simulink model "FlexibleJoint_ConventionalSMC"  (R2019b)
settings: Solver=VariableStepAuto  StartTime=0.0  StopTime=10.0  RelTol=1e-3
libraries: robotcorelib x1
settings Model: Creator=USER  LastModifiedBy=USER

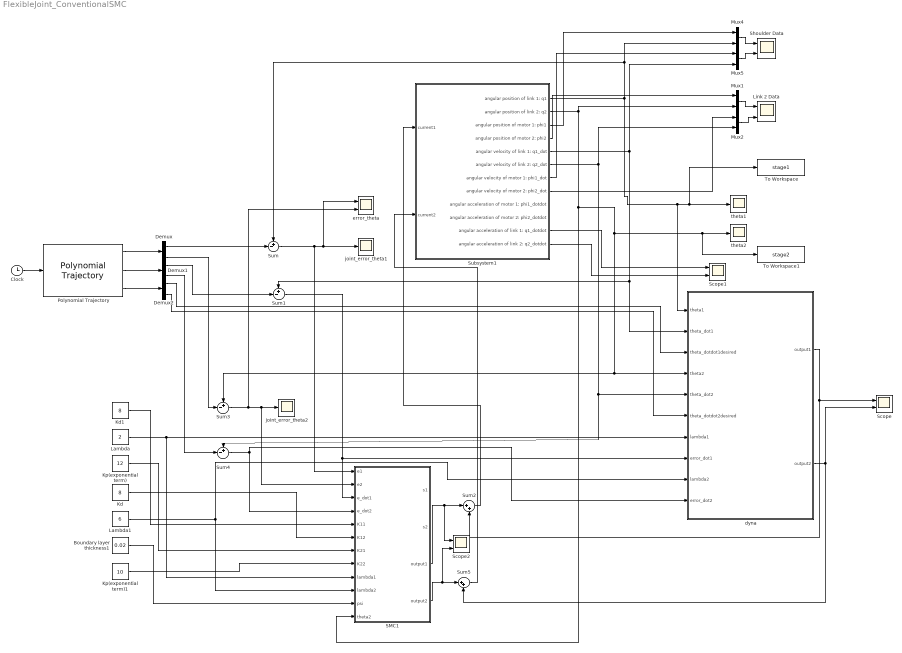
== system FlexibleJoint_ConventionalSMC ==
  Boundary layer thickness1 : Constant  Value=0.02
  Clock : Clock
  Demux : Demux  Outputs=2
  Demux1 : Demux  Outputs=2
  Demux2 : Demux  Outputs=2
  Kd : Constant  Value=8
  Kd1 : Constant  Value=8
  Kp(exponential term) : Constant  Value=12
  Kp(exponential term)1 : Constant  Value=10
  Lambda : Constant  Value=2
  Lambda1 : Constant  Value=6
  Link 2 Data : Scope  NumInputPorts=2
  Mux{1..2,4..5} (4 alike) : Mux  Inputs=2
  Polynomial Trajectory : robotcorelib/Polynomial Trajectory  WaypointSource=Internal  Waypoints=[ 0, pi/2; 0, pi/4]  TimePoints=[ 0, 5]  TimeInterval=[ 1, 4 ]  Method=Cubic Polynomial  ParameterSource=Internal  VelocityBoundaryCondition=zeros( 2, 2 )  AccelerationBoundaryCondition=zeros( 2, 5 )  SimulateUsing=Interpreted execution
      settings: SourceProductName=Robotics System Toolbox  SourceProductBaseCode=RO
  SMC1 : MATLAB Function  TreatAsAtomicUnit=on
  Scope : Scope  NumInputPorts=2
  Scope1 : Scope  NumInputPorts=2
  Scope2 : Scope  NumInputPorts=2
  Shoulder Data : Scope  NumInputPorts=2
  Subsystem1 : Subsystem
  Sum{,1,3..4} (4 alike) : Sum  Inputs=+-|
  Sum2 : Sum  Inputs=|++
  Sum5 : Sum  Inputs=|++
  To Workspace : ToWorkspace  VariableName=stage1  SaveFormat=Timeseries  SampleTime=-1
  To Workspace1 : ToWorkspace  VariableName=stage2  SaveFormat=Timeseries  SampleTime=-1
  dyna : MATLAB Function  TreatAsAtomicUnit=on
  error_theta : Scope  NumInputPorts=2
  joint_error_theta1 : Scope
  joint_error_theta2 : Scope
  theta1 : Scope
  theta2 : Scope
  wires:
  Subsystem1/5(angular velocity of link 1: q1_dot) -> Mux5/2, dyna/2(theta_dot1), Sum1/1
  Boundary layer thickness1/1 -> SMC1/11(psi)
  Sum1/1 -> SMC1/3(e_dot1), dyna/8(error_dot1)
  Sum4/1 -> dyna/10(error_dot2), SMC1/4(e_dot2)
  Polynomial Trajectory/1 -> Demux/1
  Subsystem1/12(angular acceleration of link 2: q2_dotdot) -> Scope1/2
  Demux1/2 -> Sum4/2
  Kp(exponential term)1/1 -> SMC1/8(K22)
  Clock/1 -> Polynomial Trajectory/1
  SMC1/3(output1) -> Scope2/1, Sum2/1
  Demux2/1 -> dyna/3(theta_dotdot1desired)
  Kd1/1 -> SMC1/5(K11)
  Lambda1/1 -> SMC1/10(lambda2), dyna/9(lambda2)
  Sum/1 -> SMC1/1(e1), joint_error_theta1/1, error_theta/1
  Demux1/1 -> Sum1/2
  Demux2/2 -> dyna/6(theta_dotdot2desired)
  Demux/1 -> Sum/2
  SMC1/4(output2) -> Scope2/2, Sum5/1
  Kp(exponential term)/1 -> SMC1/7(K21)
  Polynomial Trajectory/2 -> Demux1/1
  Sum2/1 -> Subsystem1/1(current1)
  Lambda/1 -> SMC1/9(lambda1), dyna/7(lambda1)
  Demux/2 -> Sum3/2
  dyna/2(output2) -> Scope/2, Sum5/2
  Subsystem1/2(angular position of link 2: q2) -> To Workspace1/1, theta2/1, Sum3/1, dyna/4(theta2), SMC1/12(theta2), Mux1/2
  Subsystem1/6(angular velocity of link 2: q2_dot) -> Sum4/1, dyna/5(theta_dot2), Mux2/2
  Polynomial Trajectory/3 -> Demux2/1
  Kd/1 -> SMC1/6(K12)
  Sum3/1 -> SMC1/2(e2), joint_error_theta2/1, error_theta/2
  Subsystem1/11(angular acceleration of link 1: q1_dotdot) -> Scope1/1
  dyna/1(output1) -> Scope/1, Sum2/2
  Sum5/1 -> Subsystem1/2("current2 ")
  Subsystem1/1(angular position of link 1: q1) -> Mux4/2, Sum/1, dyna/1(theta1), To Workspace/1, theta1/1
  Mux5/1 -> Shoulder Data/2
  Mux4/1 -> Shoulder Data/1
  Mux1/1 -> Link 2 Data/1
  Mux2/1 -> Link 2 Data/2
  Subsystem1/3(angular position of motor 1: phi1) -> Mux4/1
  Subsystem1/7(angular velocity of motor 1: phi1_dot) -> Mux5/1
  Subsystem1/4(angular position of motor 2: phi2) -> Mux1/1
  Subsystem1/8(angular velocity of motor 2: phi2_dot) -> Mux2/1

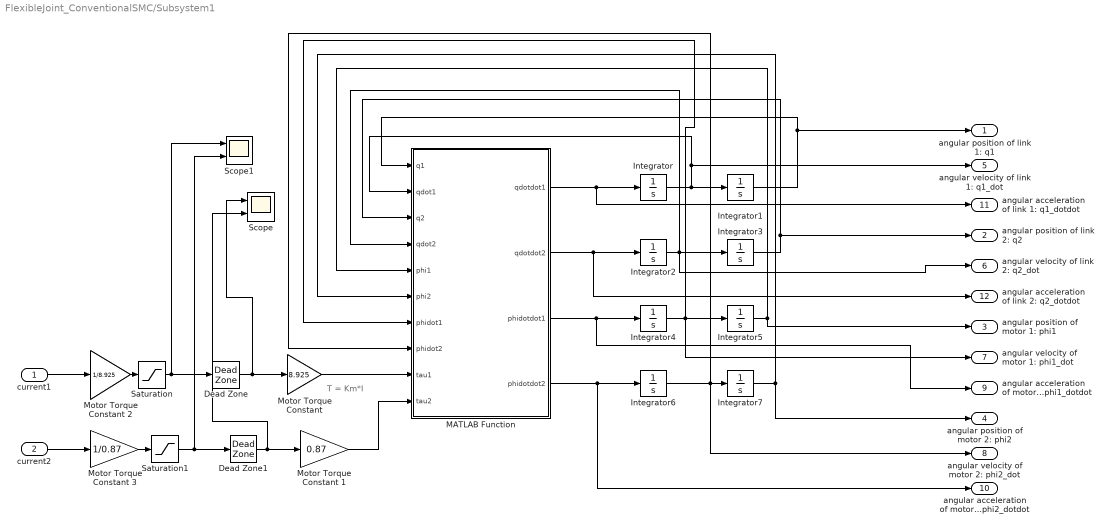
== system FlexibleJoint_ConventionalSMC/Subsystem1 ==
  note: T = Km*I
  current1 : Inport
  "current2 " : Inport  Port=2
  Dead Zone : DeadZone  LowerValue=-0.15  UpperValue=0.15  ZeroCross=off  SaturateOnIntegerOverflow=on
  Dead Zone1 : DeadZone  LowerValue=-0.15  UpperValue=0.15  ZeroCross=off  SaturateOnIntegerOverflow=on
  Integrator{,1..7} (8 alike) : Integrator
  MATLAB Function : MATLAB Function  TreatAsAtomicUnit=on
  "Motor Torque Constant " : Gain  Gain=8.925
  Motor Torque Constant 1 : Gain  Gain=0.87
  Motor Torque Constant 2 : Gain  Gain=1/8.925
  Motor Torque Constant 3 : Gain  Gain=1/0.87
  Saturation : Saturate  UpperLimit=0.94  LowerLimit=-0.94  ZeroCross=off
  Saturation1 : Saturate  ZeroCross=off
  Scope : Scope  NumInputPorts=2
  Scope1 : Scope  NumInputPorts=2
  angular position of link 1: q1 : Outport
  angular position of link 2: q2 : Outport  Port=2
  angular position of motor 1: phi1 : Outport  Port=3
  angular position of motor 2: phi2 : Outport  Port=4
  angular velocity of link 1: q1_dot : Outport  Port=5
  angular velocity of link 2: q2_dot : Outport  Port=6
  angular velocity of motor 1: phi1_dot : Outport  Port=7
  angular velocity of motor 2: phi2_dot : Outport  Port=8
  angular acceleration of motor 1: phi1_dotdot : Outport  Port=9
  angular acceleration of motor 2: phi2_dotdot : Outport  Port=10
  angular acceleration of link 1: q1_dotdot : Outport  Port=11
  angular acceleration of link 2: q2_dotdot : Outport  Port=12
  wires:
  Integrator2/1 -> angular velocity of link 2: q2_dot/1, Integrator3/1, MATLAB Function/4(qdot2)
  Integrator7/1 -> MATLAB Function/6(phi2), angular position of motor 2: phi2/1
  Integrator3/1 -> angular position of link 2: q2/1, MATLAB Function/3(q2)
  Saturation/1 -> Dead Zone/1, Scope1/1
  Integrator1/1 -> angular position of link 1: q1/1, MATLAB Function/1(q1)
  Integrator/1 -> angular velocity of link 1: q1_dot/1, MATLAB Function/2(qdot1), Integrator1/1
  Saturation1/1 -> Dead Zone1/1, Scope1/2
  Integrator6/1 -> angular velocity of motor 2: phi2_dot/1, MATLAB Function/8(phidot2), Integrator7/1
  Integrator4/1 -> angular velocity of motor 1: phi1_dot/1, Integrator5/1, MATLAB Function/7(phidot1)
  MATLAB Function/2(qdotdot2) -> angular acceleration of link 2: q2_dotdot/1, Integrator2/1
  MATLAB Function/3(phidotdot1) -> angular acceleration of motor 1: phi1_dotdot/1, Integrator4/1
  Integrator5/1 -> angular position of motor 1: phi1/1, MATLAB Function/5(phi1)
  MATLAB Function/4(phidotdot2) -> angular acceleration of motor 2: phi2_dotdot/1, Integrator6/1
  Dead Zone/1 -> "Motor Torque Constant "/1, Scope/1
  MATLAB Function/1(qdotdot1) -> angular acceleration of link 1: q1_dotdot/1, Integrator/1
  Dead Zone1/1 -> Motor Torque Constant 1/1, Scope/2
  "Motor Torque Constant "/1 -> MATLAB Function/9(tau1)
  Motor Torque Constant 1/1 -> MATLAB Function/10(tau2)
  current1/1 -> Motor Torque Constant 2/1
  "current2 "/1 -> Motor Torque Constant 3/1
  Motor Torque Constant 2/1 -> Saturation/1
  Motor Torque Constant 3/1 -> Saturation1/1

== matlab function FlexibleJoint_ConventionalSMC/dyna ==
  data: theta1 input; output1 output; theta_dot1 input; theta_dotdot1desired input; theta2 input; theta_dot2 input; theta_dotdot2desired input; lambda1 input; error_dot1 input; lambda2 input; error_dot2 input; output2 output
function [output1, output2] = dyna(theta1, theta_dot1, theta_dotdot1desired, theta2, theta_dot2, theta_dotdot2desired, lambda1, error_dot1, lambda2, error_dot2)

m1 =  1.51 ; 
m2 = 0.87326;
L1 = 0.343;
L2 = 0.267;
Lc1 = 0.1590;
Lc2 = 0.0550;
I1 = 0.0392;
I2 = 0.0081;
B1 = 0.070364;
B2 = 0.028211;

% m1 = 0.5; 
% m2 = 1;
% L1 = 0.343;
% L2 = 0.267;
% Lc1 = 0.2;
% Lc2 = 0.25;
% I1 = 0.01;
% I2 = 0.01;
% B1 = 0.070364;
% B2 = 0.028211;
    
output1 = (theta_dotdot2desired - error_dot2*lambda2)*(m2*Lc2^2 + L1*m2*cos(theta2)*Lc2 + I2) - theta_dot2*(L1*Lc2*theta_dot1*m2*sin(theta2) + L1*Lc2*theta_dot2*m2*sin(theta2)) + B1*theta_dot1 + (theta_dotdot1desired - error_dot1*lambda1)*(I1 + I2 + m2*(L1^2 + 2*cos(theta2)*L1*Lc2 + Lc2^2) + Lc1^2*m1) - L1*Lc2*theta_dot1*theta_dot2*m2*sin(theta2);
output2 = L1*Lc2*m2*sin(theta2)*theta_dot1^2 + (theta_dotdot2desired - error_dot2*lambda2)*(m2*Lc2^2 + I2) + (theta_dotdot1desired - error_dot1*lambda1)*(m2*Lc2^2 + L1*m2*cos(theta2)*Lc2 + I2) + B2*theta_dot2;

end

== matlab function FlexibleJoint_ConventionalSMC/SMC1 ==
  data: s1 output; s2 output; e1 input; output1 output; e2 input; e_dot1 input; e_dot2 input; K11 input; K12 input; K21 input; K22 input; lambda1 input; lambda2 input; psi input; output2 output; theta2 input
function [s1,s2,output1, output2] = smc(e1, e2, e_dot1, e_dot2, K11, K12, K21, K22, lambda1, lambda2, psi, theta2)
    s1 = lambda1 * e1 + e_dot1;
    s2 = lambda2 * e2 + e_dot2;
         
    m1 =  1.51 ; 
    m2 = 0.87326;
    L1 = 0.343;
    L2 = 0.267;
    Lc1 = 0.1590;
    Lc2 = 0.0550;
    I1 = 0.0392;
    I2 = 0.0081;
    B1 = 0.070364;
    B2 = 0.028211;
    
    if (abs(s1) > psi)    
        sat_s1 = sign(s1);
    else
        sat_s1 = s1/psi;
    end
    
    if (abs(s2) > psi)    
        sat_s2 = sign(s2);
    else
        sat_s2 = s2/psi;
    end
    
%     output = (-Kd * sat_s - Kp*s)/(m2*Lc2^2 + I2);
    output1 = (-K21 * sat_s2 - K22*s2)*(m2*Lc2^2 + L1*m2*cos(theta2)*Lc2 + I2) + (-K11 * sat_s1 - K12*s1)*(I1 + I2 + m2*(L1^2 + 2*cos(theta2)*L1*Lc2 + Lc2^2) + Lc1^2*m1);
    output2 = (-K11 * sat_s1 - K12*s1)*(m2*Lc2^2 + L1*m2*cos(theta2)*Lc2 + I2) + (-K21 * sat_s2 - K22*s2)*(m2*Lc2^2 + I2);
end

== matlab function FlexibleJoint_ConventionalSMC/Subsystem1/MATLAB Function ==
  data: q1 input; qdotdot1 output; qdot1 input; q2 input; qdot2 input; phi1 input; phi2 input; phidot1 input; phidot2 input; tau1 input; tau2 input; qdotdot2 output; phidotdot1 output; phidotdot2 output
function [qdotdot1,qdotdot2,phidotdot1,phidotdot2] = fcn(q1,qdot1,q2,qdot2,phi1,phi2,phidot1,phidot2,tau1,tau2)
%y is thetadotdot
tau = [0;0;tau1;tau2];
%Veltman Thesis Values
% m1 = 0.5; 
% m2 = 1;
% L1 = 0.343;
% L2 = 0.267;
% Lc1 = 0.2;
% Lc2 = 0.25;
% I1 = 0.01;
% I2 = 0.01;
% B1 = 0.070364;
% B2 = 0.028211;

%Electrical School values
L1 = 0.343;
L2 = 0.267;
Lc1 = 0.1590;
Lc2 = 0.0550;
m1 = 1.51;
m2 = 0.87326;
I1 = 0.0392;
I2 = 0.0081;
B1 = 0.070364;
B2 = 0.028211;
Bm1 =4.5;
Bm2 = 0.5;
Ks1 = 9;
Ks2 = 4;
Ir1 = 0.0628;
Ir2 = 0.0026;

z = [0 0;
     0 0];
M11 = I2+I1+m2*((L1^2)+(Lc2^2)+2*L1*Lc2*cos(q2))+m1*(Lc1^2);
M12 = I2+m2*(Lc2^2)+L1*Lc2*m2*cos(q2);
M21 = M12;
M22 = I2+m2*(Lc2^2);

M1 = [M11 M12;
     M21 M22];

M2 = [Ir1 0;
      0 Ir2];
  
M = [M1 z;
     z  M2];
 
C11 = -m2*L1*Lc2*sin(q2)*qdot2;
C12 = -m2*L1*Lc2*sin(q2)*qdot2-m2*L1*Lc2*sin(q2)*qdot1;
C21 = m2*L1*Lc2*sin(q2)*qdot1;
C22 = 0;

Ca = [C11 C12;
     C21 C22];

C = [Ca z;
     z  z];
 
K1 = [Ks1 0;
      0  Ks2];
  
K = [K1 -K1;
     -K1 K1];
 
fvl = [B1 0;
      0  B2];
  
fvm = [Bm1 0;
       0  Bm2];
   
fv = [fvl z;
      z  fvm];
  
fvf = fv*[qdot1;qdot2;phidot1;phidot2];
Cf = C*[qdot1;qdot2;phidot1;phidot2];
Kf = K*[q1;q2;phi1;phi2];

y = inv(M)*(tau-Cf-fvf-Kf);
qdotdot1 = y(1);
qdotdot2 = y(2);
phidotdot1 = y(3);
phidotdot2 = y(4);
